simulink model "Project1_3"  (R2017a)
settings: Solver=ode45  StartTime=0.0  StopTime=1  MaxStep=1e-4  RelTol=1e-3
values from neighbouring files (symbols this model uses):
  ki = ac^2*L    [Project1Var.m]
  kp = ac*L    [Project1Var.m]
  L = 2.5*10^(-3)    (= 0.0025)    [Project1Var.m]
  psi = 0.35    [Project1Var.m]
  R = 0.5    [Project1Var.m]
  Vn = 120    [Project1Var.m]
undefined symbols (not defined in the file): Ra
settings Model: Creator=Callum  LastModifiedBy=Callum

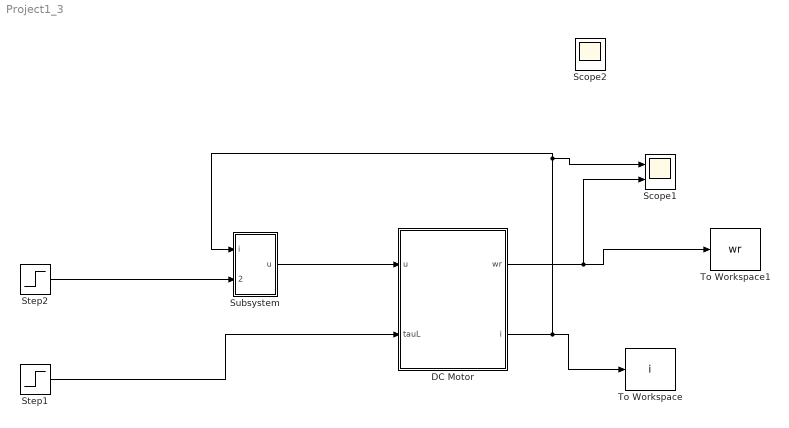
== system Project1_3 ==
  DC Motor : Subsystem  mask{R=R, L=L, psi=psi, J=0.1}
      mask prompts: R "R (ohm)"; L "L (H)"; psi "psi(Vs)"; J "J (kgm^2)"
  Scope1 : Scope  NumInputPorts=2
  Scope2 : Scope
  Step1 : Step  Time=0.3  After=7  SampleTime=0
  Step2 : Step  Time=0.1  After=20  SampleTime=0
  Subsystem : Subsystem  mask{kp=kp, ki=ki, Rab=Ra}
      mask prompts: Rab "Ra"
  To Workspace : ToWorkspace  VariableName=i  SaveFormat=Timeseries  SampleTime=-1
      settings: Save2DSignal=2-D array (concatenate along first dimension)
  To Workspace1 : ToWorkspace  VariableName=wr  SaveFormat=Timeseries  SampleTime=-1
      settings: Save2DSignal=2-D array (concatenate along first dimension)
  wires:
  DC Motor/2(i) -> Scope1/1, Subsystem/1(i), To Workspace/1
  DC Motor/1(wr) -> Scope1/2, To Workspace1/1
  Step1/1 -> DC Motor/2(tauL)
  Subsystem/1(u) -> DC Motor/1(u)
  Step2/1 -> Subsystem/2(i_ref)

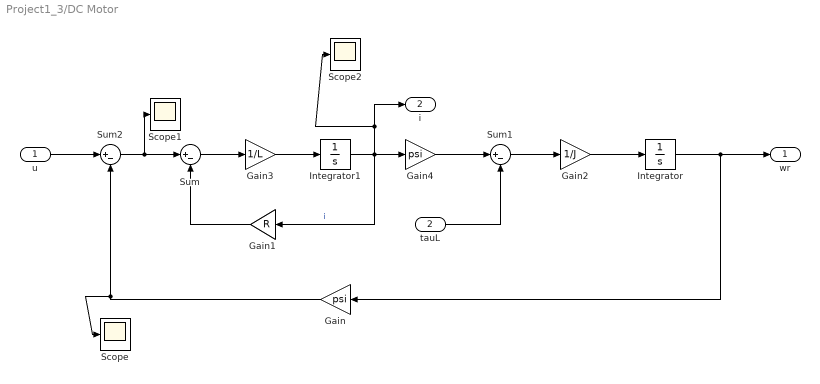
== system Project1_3/DC Motor ==
  u : Inport
  tauL : Inport  Port=2
  Gain : Gain  Gain=psi
  Gain1 : Gain  Gain=R
  Gain2 : Gain  Gain=1/J
  Gain3 : Gain  Gain=1/L
  Gain4 : Gain  Gain=psi
  Integrator : Integrator
  Integrator1 : Integrator
  Scope : Scope
  Scope1 : Scope
  Scope2 : Scope
  Sum : Sum  Inputs=|+-
  Sum1 : Sum  Inputs=|+-
  Sum2 : Sum  Inputs=|+-
  wr : Outport
  i : Outport  Port=2
  wires:
  u/1 -> Sum2/1
  Integrator1/1 -> Scope2/1, i/1, Gain1/1, Gain4/1  "i"
  Gain/1 -> Scope/1, Sum2/2
  tauL/1 -> Sum1/2
  Gain4/1 -> Sum1/1
  Integrator/1 -> wr/1, Gain/1
  Sum1/1 -> Gain2/1
  Gain2/1 -> Integrator/1
  Sum/1 -> Gain3/1
  Sum2/1 -> Scope1/1, Sum/1
  Gain3/1 -> Integrator1/1
  Gain1/1 -> Sum/2

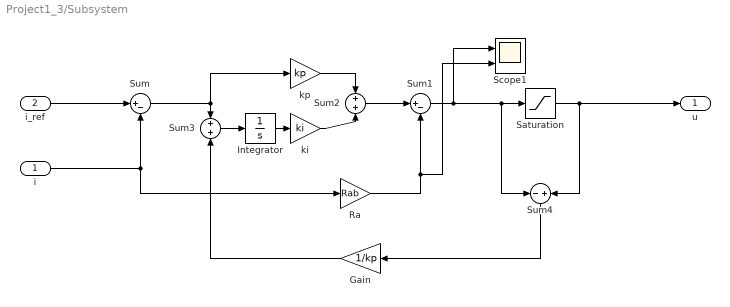
== system Project1_3/Subsystem ==
  i : Inport
  i_ref : Inport  Port=2
  Gain : Gain  Gain=1/kp
  Integrator : Integrator
  Ra : Gain  Gain=Rab
  Saturation : Saturate  UpperLimit=Vn  LowerLimit=-Vn
  Scope1 : Scope  NumInputPorts=2
  Sum : Sum  Inputs=|+-
  Sum1 : Sum  Inputs=|+-
  Sum2 : Sum
  Sum3 : Sum
  Sum4 : Sum  Inputs=-+
  ki : Gain  Gain=ki
  kp : Gain  Gain=kp
  u : Outport
  wires:
  Sum2/1 -> Sum1/1
  Sum1/1 -> Scope1/1, Sum4/1, Saturation/1
  Ra/1 -> Scope1/2, Sum1/2
  kp/1 -> Sum2/1
  i/1 -> Ra/1, Sum/2
  i_ref/1 -> Sum/1
  Integrator/1 -> ki/1
  Saturation/1 -> Sum4/2, u/1
  Sum3/1 -> Integrator/1
  Sum4/1 -> Gain/1
  Sum/1 -> Sum3/1, kp/1
  ki/1 -> Sum2/2
  Gain/1 -> Sum3/2
